simulink model "multistageNLMPC_controlBlock_withIntegralControl_mdlRef"  (R2024b)
settings: Solver=FixedStepAuto  StartTime=0.0  StopTime=inf  RelTol=1e-3
values from neighbouring files (symbols this model uses):
  predHorizon = pvstage(2)    [MyNMPC.m]    (also in NonlinearSystemControl_withKoopman_and_nlmpcMultistage.m = 10)
  pvcost = [current_ref; predHorizon; Q; R; S; Qi]    [NonlinearSystemControl_withKoopman_and_nlmpcMultistage.m]
  u0 = zeros(nu,1)    [NonlinearSystemControl_withKoopman_and_nlmpcMultistage.m]
libraries: mpclib x1
settings Model: Creator=fnae  LastModifiedBy=fnae
settings RTWCC: GPUComputeCapability=3.5

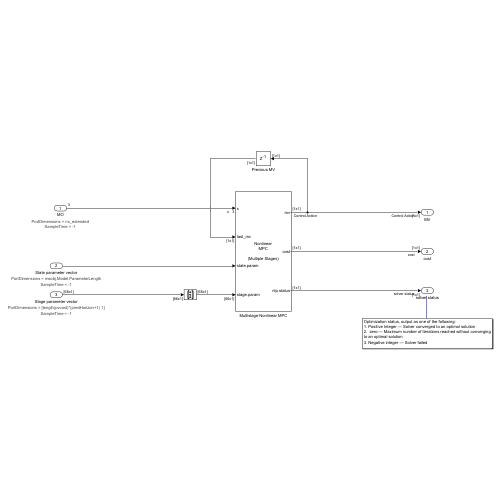
[thumbnail: Simulink's stored preview of the top-level diagram]
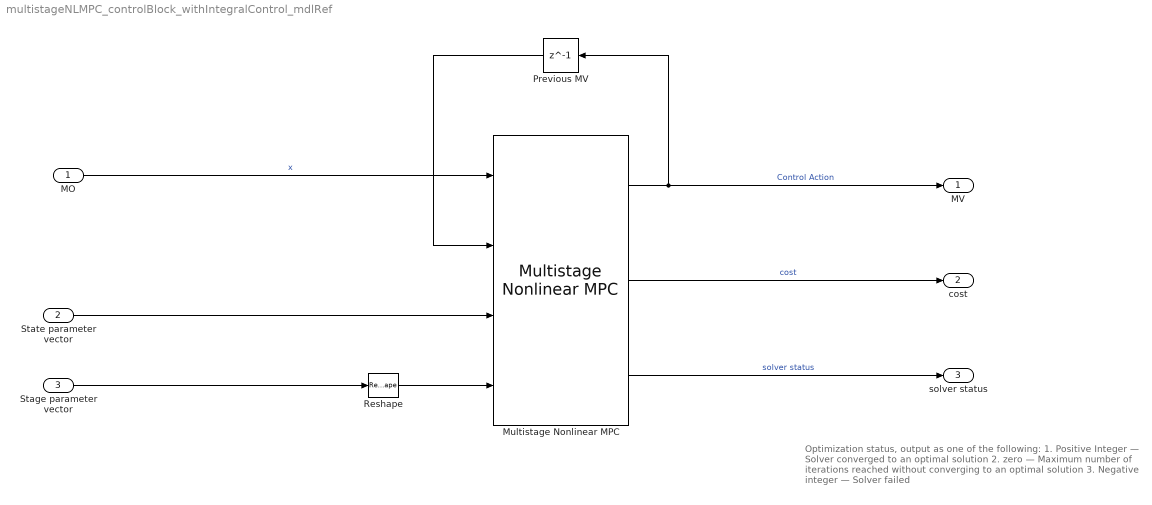
== system multistageNLMPC_controlBlock_withIntegralControl_mdlRef ==
  note: Optimization status, output as one of the following:
      | 1. Positive Integer — Solver converged to an optimal solution
      | 2.  zero — Maximum number of iterations reached without converging to an optimal solution
      | 3. Negative integer — Solver failed
  MO : Inport  PortDimensions=nx_extended
      settings: AttributesFormatString=|
      | PortDimensions = %<PortDimensions>
      | SampleTime = %<SampleTime>
  State parameter vector : Inport  Port=2  PortDimensions=msobj.Model.ParameterLength
      settings: AttributesFormatString=|
      | PortDimensions = %<PortDimensions>
      | SampleTime = %<SampleTime>
  Stage parameter vector : Inport  Port=3  PortDimensions=[length(pvcost)*(predHorizon+1) 1]
      settings: AttributesFormatString=|
      | PortDimensions = %<PortDimensions>
      | SampleTime = %<SampleTime>
  Multistage Nonlinear MPC : mpclib/Multistage Nonlinear MPC  nlmpcobj=msobj  UseObjectTs=on  TsControl=-1  UseMEX=on  mexname=nlmpcControllerMEX_withIntegralControl  md_enabled=off  stateparam_enabled=on  stageparam_enabled=on  cost_enabled=on  mvseq_enabled=off  stateseq_enabled=off  slack_enabled=off  status_enabled=on  mv_min=off  mv_max=off  mvrate_min=off  mvrate_max=off  state_min=off  state_max=off  terminal_state=off  nlp_initialize=off
  Previous MV : Delay  DelayLength=1  InitialCondition=u0
  Reshape : Reshape  OutputDimensionality=Column vector (2-D)
  MV : Outport
  cost : Outport  Port=2
  solver status : Outport  Port=3
  wires:
  Multistage Nonlinear MPC/1 -> MV/1, Previous MV/1  "Control Action"
  Multistage Nonlinear MPC/2 -> cost/1  "cost"
  MO/1 -> Multistage Nonlinear MPC/1  "x"
  Multistage Nonlinear MPC/3 -> solver status/1  "solver status"
  Previous MV/1 -> Multistage Nonlinear MPC/2
  Reshape/1 -> Multistage Nonlinear MPC/4
  Stage parameter vector/1 -> Reshape/1
  State parameter vector/1 -> Multistage Nonlinear MPC/3
